simulink model "spiral1"  (R2024b)
settings: Solver=FixedStepAuto  StartTime=0.0  StopTime=inf  FixedStep=0.05  RelTol=1e-3
undefined symbols (not defined in the file): angular, linear
libraries: ros2lib x3
settings Model: Creator=advance_control_lab  LastModifiedBy=advance_control_lab
settings OptimizationCC: DefaultParameterBehavior=Inlined  EnhancedBackFolding=on  PassReuseOutputArgsAs=Individual arguments  ZeroExternalMemoryAtStartup=off  ZeroInternalMemoryAtStartup=off  MaxStackSize=64  OptimizeBlockOrder=speed  DifferentSizesBufferReuse=on  OptimizationCustomize=off  EfficientTunableParamExpr=on
settings DebuggingCC: ParameterTunabilityLossMsg=error
settings HardwareCC: ProdBitPerLong=64  ProdHWDeviceType=Intel->x86-64 (Linux 64)
settings SFSimCC: MATLABDynamicMemAlloc=off
settings RTWCC: Description=Embedded Coder  SystemTargetFile=ert.tlc  HardwareBoard=Robot Operating System 2 (ROS 2)  TLCOptions="-aInlineSetEventsForThisBaseRateFcn=TLC_FALSE -aSuppressMultiTaskScheduler=TLC_FALSE  -aRateBasedStepFcn=0"  GenCodeOnly=on  TemplateMakefile=ert_default_tmf  Toolchain=Colcon Tools  TargetLang=C++
settings CodeAppCC: ForceParamTrailComments=on  IgnoreCustomStorageClasses=off  OperatorAnnotations=on  SimulinkDataObjDesc=on  SFDataObjDesc=on  InsertBlockDesc=on
settings ERTTargetCC: CodeInterfacePackaging=C++ class  SupportVariableSizeSignals=on  RootIOFormat=Structure reference

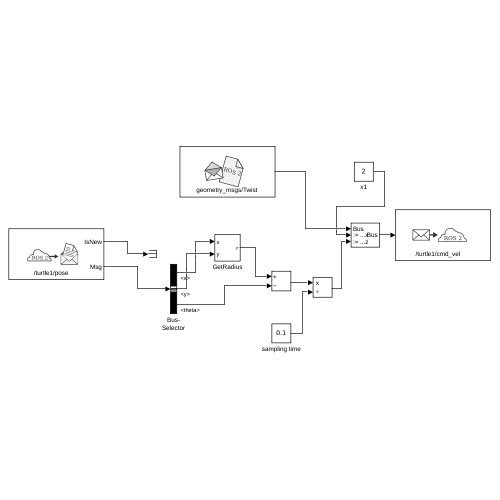
[thumbnail: Simulink's stored preview of the top-level diagram]
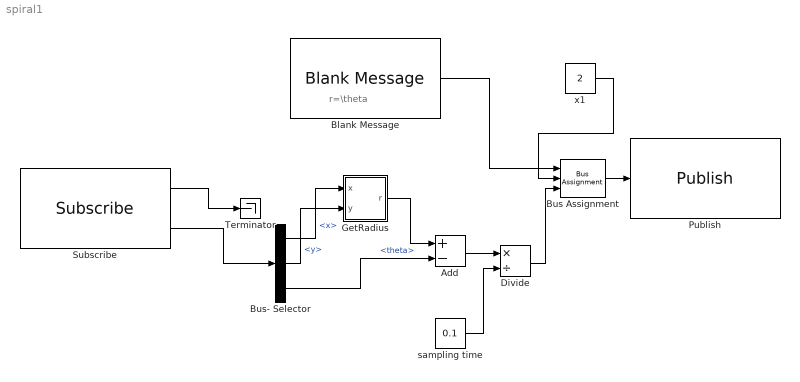
== system spiral1 ==
  note: r=\theta
  Add : Sum  Inputs=+-
  Blank Message : ros2lib/Blank Message  messageClass=Message  entityType=geometry_msgs/Twist  messageType=geometry_msgs/Twist  SampleTime=inf
  Bus Assignment : BusAssignment  AssignedSignals=linear.x,angular.z
  Bus- Selector : BusSelector  OutputSignals=x,y,theta
  Divide : Product  Inputs=*/
  GetRadius : Subsystem
  Publish : ros2lib/Publish  topicSource=Select from ROS network  topic=/turtle1/cmd_vel  messageType=geometry_msgs/Twist  QOSHistory=Keep last  QOSDepth=1  QOSReliability=Reliable  QOSDurability=Volatile  QOSDeadline=Inf  QOSLifespan=Inf  QOSLiveliness=Automatic  QOSLeaseDuration=Inf  QOSAvoidROSNamespaceConventions=off
  Subscribe : ros2lib/Subscribe  topicSource=Specify your own  topic=/turtle1/pose  messageType=geometry_msgs/Pose2D  sampleTime=-1  QOSHistory=Keep last  QOSDepth=1  QOSReliability=Reliable  QOSDurability=Volatile  QOSDeadline=Inf  QOSLifespan=Inf  QOSLiveliness=Automatic  QOSLeaseDuration=Inf  QOSAvoidROSNamespaceConventions=off
  Terminator : Terminator
  sampling time : Constant  Value=0.1
  x1 : Constant  Value=2
  wires:
  Subscribe/1 -> Terminator/1
  Subscribe/2 -> Bus- Selector/1
  Blank Message/1 -> Bus Assignment/1
  Bus Assignment/1 -> Publish/1
  x1/1 -> Bus Assignment/2
  GetRadius/1(r) -> Add/1
  Add/1 -> Divide/1
  sampling time/1 -> Divide/2
  Divide/1 -> Bus Assignment/3
  Bus- Selector/3 -> Add/2  "<theta>"
  Bus- Selector/1 -> GetRadius/1(x)  "<x>"
  Bus- Selector/2 -> GetRadius/2(y)  "<y>"

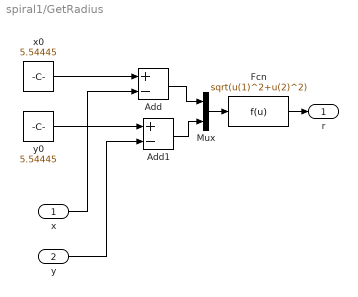
== system spiral1/GetRadius ==
  x : Inport
  y : Inport  Port=2
  Add : Sum  Inputs=+-
  Add1 : Sum  Inputs=+-
  Fcn : Fcn  Expr=sqrt(u(1)^2+u(2)^2)
  Mux : Mux  Inputs=2
  x0 : Constant  Value=5.54445
  y0 : Constant  Value=5.54445
  r : Outport
  wires:
  Add1/1 -> Mux/2
  Add/1 -> Mux/1
  Mux/1 -> Fcn/1
  x0/1 -> Add/1
  y0/1 -> Add1/1
  Fcn/1 -> r/1
  y/1 -> Add1/2
  x/1 -> Add/2
